simulink model "rfsoc4x2_tut_rfdc"  (R2019a)
settings: Solver=VariableStepAuto  StartTime=0.0  StopTime=10.0  RelTol=1e-3
undefined symbols (not defined in the file): I, Q
libraries: xbsIndex_r4 x704, casper_library_misc x5, xps_library x1
(part 1 of 14)
settings Model: Creator=mcb  LastModifiedBy=mcb

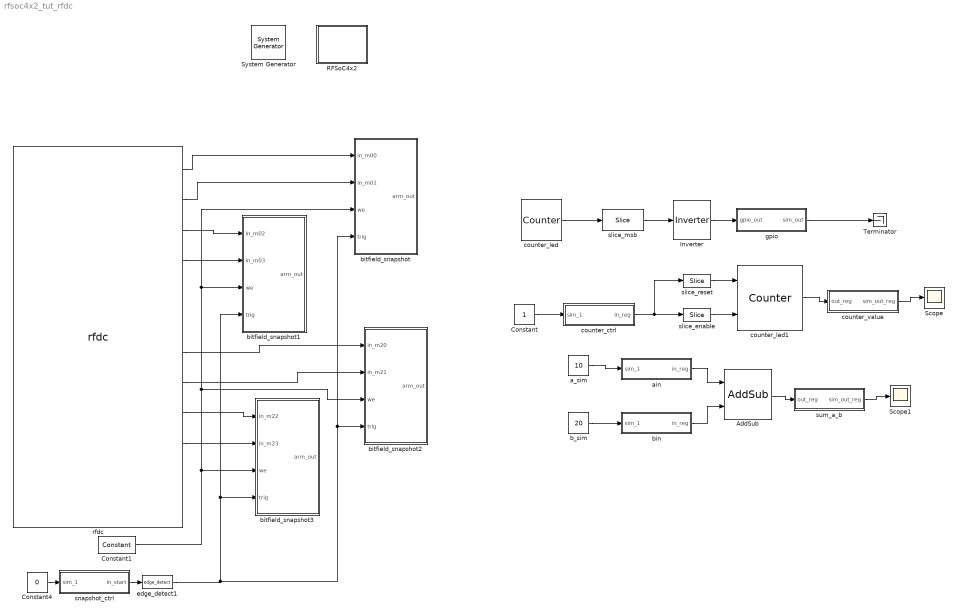
== system rfsoc4x2_tut_rfdc ==
  " System Generator" : xbsIndex_r4/ System Generator  Tag=genX  xilinxfamily=zynquplusRFSOC  part=xczu48dr  speed=-2-e  package=ffvg1517  synthesis_tool=XST  clock_wrapper=Clock Enables  directory=/home/mcb/git/casper/tutorials_devel/rfsoc/tut_rfdc/rfsoc4x2_tut_rfdc/sysgen  proj_type=Vivado  Synth_file=Vivado Synthesis Defaults  Impl_file=Vivado Implementation Defaults  testbench=off  simulink_period=1  sysclk_period=4.069  dcm_input_clock_period=10  incr_netlist=off  trim_vbits=Everywhere in SubSystem  dbl_ovrd=According to Block Masks  core_generation=According to Block Masks  run_coregen=off  deprecated_control=off  eval_field=0  block_type=sysgen
  AddSub : xbsIndex_r4/AddSub  mode=Addition  use_carryin=off  use_carryout=off  en=off  latency=0  precision=User Defined  arith_type=Unsigned  n_bits=32  bin_pt=0  quantization=Truncate  overflow=Saturate  use_behavioral_HDL=off  hw_selection=Fabric  pipelined=off  dbl_ovrd=off  block_type=addsub
  Constant : Constant
  Constant1 : xbsIndex_r4/Constant  const=1.0  gui_display_data_type=Boolean  arith_type=Boolean  n_bits=16  bin_pt=14  preci_type=Single  exp_width=8  frac_width=24  explicit_period=on  period=1  equ=P=C  opselect=C  inp2=PCIN>>17  opr=+  inp1=P  carry=CIN  dbl_ovrd=off  block_type=constant
  Constant4 : Constant  Value=0
  Inverter : xbsIndex_r4/Inverter  en=off  latency=0  dbl_ovrd=off  block_type=inv
  RFSoC4x2 : Subsystem  Tag=xps:xsg  AncestorBlock=xps_library/Platforms/ZCU216  mask(xsg core config){hw_sys=rfsoc4x2:xczu48dr, clk_src=adc_clk, clk_rate=245.76, pl_clk_rate=122.88, sample_period=1, synthesis_tool=XST}
      mask prompts: hw_sys "Hardware Platform"; clk_src "User IP Clock source"; clk_rate "User IP Clock Rate (MHz)"; pl_clk_rate "RFPLL PL Clock Rate (MHz)"; sample_period "Sample Period"; synthesis_tool "Synthesis Tool:"
      mask help:
      | The XSG Core Config block is used to configure the System Generator design
      | for the casper_xps toolflow. Settings here are used to configure the
      | Xilinx System Generator block parameters automatically, and control toolflow
      | script  execution. It needs to be at the top level of all designs being compiled
      | with the casper_xps toolflow.
      mask init:
      | xps_xsg_rfsoc4x2_conf_mask;
      mask Help: eval('xlWeb([getenv(''MLIB_ROOT''), ''\doc\html\sys_xsg_core_config\sys_xsg_core_config.html''])')
      mask TypeOptions hw_sys: rfsoc4x2:xczu48dr
      mask TypeOptions clk_src: adc_clk
      mask TypeOptions synthesis_tool: Leonardo Spectrum | Synplify | Synplify Pro | XST
      mask Display: fprintf(['RFSoC4x2']);
  Scope : Scope
  Scope1 : Scope
  Terminator : Terminator
  a_sim : Constant  Value=10
  ain : Subsystem  Tag=xps:sw_reg  AncestorBlock=xps_library/Memory/software_register  mask(swreg){io_dir=From Processor, io_delay=0, init_val=0, sample_period=1, names=reg, bitwidths=32, bin_pts=0, arith_types=0, sim_port=on, show_format=off}
      mask prompts: io_dir "I/O direction"; io_delay "I/O delay"; init_val "Initial Value"; sample_period "Sample period"; names "Bitfield names [msb...lsb]"; bitwidths "Bitfield widths"; bin_pts "Bitfield binary pts"; arith_types "Bitfield types, ufix=0, fix=1, bool=2"; sim_port "Provide sim input/output?"; show_format "Print format string?"
      mask help: A 32-bit software-accessible register. Can be divided into bitfields of varying widths and types using the fields in the block mask.
      mask init:
      | swreg_init(gcb)
      settings: AttributesFormatString=1input
      mask TypeOptions io_dir: To Processor | From Processor
      mask Callback io_dir:
      | mask_enables = get_param(gcb, 'MaskEnables');
      | mask_names = get_param(gcb, 'MaskNames');
      | if strcmp(get_param(gcb, 'io_dir'), 'To Processor'),
      |     mask_enables{ismember(mask_names, 'sample_period')} = 'off';
      | else
      |     mask_enables{ismember(mask_names, 'sample_period')} = 'on';
      | end
      | set_param(gcb, 'MaskEnables', mask_enables);
      mask DialogControl ParameterTabVar0 Prompt: Setup
  b_sim : Constant  Value=20
  bin : Subsystem  Tag=xps:sw_reg  AncestorBlock=xps_library/Memory/software_register  mask(swreg){io_dir=From Processor, io_delay=0, init_val=0, sample_period=1, names=reg, bitwidths=32, bin_pts=0, arith_types=0, sim_port=on, show_format=off}
      mask prompts: io_dir "I/O direction"; io_delay "I/O delay"; init_val "Initial Value"; sample_period "Sample period"; names "Bitfield names [msb...lsb]"; bitwidths "Bitfield widths"; bin_pts "Bitfield binary pts"; arith_types "Bitfield types, ufix=0, fix=1, bool=2"; sim_port "Provide sim input/output?"; show_format "Print format string?"
      mask help: A 32-bit software-accessible register. Can be divided into bitfields of varying widths and types using the fields in the block mask.
      mask init:
      | swreg_init(gcb)
      settings: AttributesFormatString=1input
      mask TypeOptions io_dir: To Processor | From Processor
      mask Callback io_dir:
      | mask_enables = get_param(gcb, 'MaskEnables');
      | mask_names = get_param(gcb, 'MaskNames');
      | if strcmp(get_param(gcb, 'io_dir'), 'To Processor'),
      |     mask_enables{ismember(mask_names, 'sample_period')} = 'off';
      | else
      |     mask_enables{ismember(mask_names, 'sample_period')} = 'on';
      | end
      | set_param(gcb, 'MaskEnables', mask_enables);
      mask DialogControl ParameterTabVar0 Prompt: Setup
  bitfield_snapshot : Subsystem  Tag=casper:bitsnap  AncestorBlock=casper_library_scopes/bitfield_snapshot  mask(bitsnap){io_names=[m00, m01], io_widths=[64 64], io_bps=[0 0], io_types=[1 1], show_format=on, snap_storage=bram, snap_dram_dimm=2, snap_dram_clock=250, snap_nsamples=14, snap_data_width=128, snap_offset=off, snap_circap=off, snap_value=off, snap_ext_arm=off, snap_ext_circ=off, snap_provide_outputs=on, snap_use_dsp48=on, snap_delay=2, extra_names=[c d], extra_widths=[30 2], extra_bps=[0 0], extra_types=[0 0]}
      mask prompts: io_names "Names [msb...lsb]"; io_widths "Bitwidths [msb...lsb]"; io_bps "Binary pts [msb...lsb]"; io_types "Data types [msb...lsb], ufix=0, fix=1, bool=2"; show_format "Print format string?"; snap_storage "Storage medium"; snap_dram_dimm "DRAM dimm"; snap_dram_clock "DRAM clock rate"; snap_nsamples "Number of Samples (2^?)"; snap_data_width "Data width"; snap_offset "Start delay support"; snap_circap "Circular capture support"; snap_value "Extra value capture support"; snap_ext_arm "External arm support"; snap_ext_circ "External circular capture support"; snap_provide_outputs "Provide outputs"; snap_use_dsp48 "Use DSP48s to implement counters"; snap_delay "Pre-snapshot delay"; extra_names "Names [msb...lsb]"; extra_widths "Widths [msb...lsb]"; extra_bps "Binary pts [msb...lsb]"; extra_types "Data types [msb...lsb], ufix=0, fix=1, bool=2"
      mask help:
      | A wrapped snapshot block. Allows specification of inputs to a snapblock word so the toolflow can automatically set up the scope.
      | See documentation for snapshot for explanation of parameters.
      mask init:
      | bitsnap_init(gcb);
      settings: AttributesFormatString=|
      | snap(2):f64.0,f64.0 = 128 bits\n128 wide, 16384 deep
      | debugID: 67280215
      mask TypeOptions snap_storage: bram | dram
      mask Callback snap_storage: bitsnap_callback();
      mask TypeOptions snap_dram_dimm: 1 | 2 | 3 | 4
      mask TypeOptions snap_dram_clock: 200 | 250 | 266 | 300 | 333
      mask TypeOptions snap_data_width: 8 | 16 | 32 | 64 | 128
      mask Callback snap_value: bitsnap_callback();
      mask Callback snap_ext_arm: bitsnap_callback();
      mask Callback snap_ext_circ: bitsnap_callback();
      mask Callback snap_provide_outputs: bitsnap_callback();
      mask DialogControl ParameterTabVar0 Prompt: Inputs
      mask DialogControl ParameterTabVar01 Prompt: Snapshot
      mask DialogControl ParameterTabVar012 Prompt: Extra Value
  bitfield_snapshot1 : Subsystem  Tag=casper:bitsnap  AncestorBlock=casper_library_scopes/bitfield_snapshot  mask(bitsnap){io_names=[m02, m03], io_widths=[64 64], io_bps=[0 0], io_types=[1 1], show_format=on, snap_storage=bram, snap_dram_dimm=2, snap_dram_clock=250, snap_nsamples=14, snap_data_width=128, snap_offset=off, snap_circap=off, snap_value=off, snap_ext_arm=off, snap_ext_circ=off, snap_provide_outputs=on, snap_use_dsp48=on, snap_delay=2, extra_names=[c d], extra_widths=[30 2], extra_bps=[0 0], extra_types=[0 0]}
      mask prompts: io_names "Names [msb...lsb]"; io_widths "Bitwidths [msb...lsb]"; io_bps "Binary pts [msb...lsb]"; io_types "Data types [msb...lsb], ufix=0, fix=1, bool=2"; show_format "Print format string?"; snap_storage "Storage medium"; snap_dram_dimm "DRAM dimm"; snap_dram_clock "DRAM clock rate"; snap_nsamples "Number of Samples (2^?)"; snap_data_width "Data width"; snap_offset "Start delay support"; snap_circap "Circular capture support"; snap_value "Extra value capture support"; snap_ext_arm "External arm support"; snap_ext_circ "External circular capture support"; snap_provide_outputs "Provide outputs"; snap_use_dsp48 "Use DSP48s to implement counters"; snap_delay "Pre-snapshot delay"; extra_names "Names [msb...lsb]"; extra_widths "Widths [msb...lsb]"; extra_bps "Binary pts [msb...lsb]"; extra_types "Data types [msb...lsb], ufix=0, fix=1, bool=2"
      mask help:
      | A wrapped snapshot block. Allows specification of inputs to a snapblock word so the toolflow can automatically set up the scope.
      | See documentation for snapshot for explanation of parameters.
      mask init:
      | bitsnap_init(gcb);
      settings: AttributesFormatString=|
      | snap(2):f64.0,f64.0 = 128 bits\n128 wide, 16384 deep
      | debugID: 72415094
      mask TypeOptions snap_storage: bram | dram
      mask Callback snap_storage: bitsnap_callback();
      mask TypeOptions snap_dram_dimm: 1 | 2 | 3 | 4
      mask TypeOptions snap_dram_clock: 200 | 250 | 266 | 300 | 333
      mask TypeOptions snap_data_width: 8 | 16 | 32 | 64 | 128
      mask Callback snap_value: bitsnap_callback();
      mask Callback snap_ext_arm: bitsnap_callback();
      mask Callback snap_ext_circ: bitsnap_callback();
      mask Callback snap_provide_outputs: bitsnap_callback();
      mask DialogControl ParameterTabVar0 Prompt: Inputs
      mask DialogControl ParameterTabVar01 Prompt: Snapshot
      mask DialogControl ParameterTabVar012 Prompt: Extra Value
  bitfield_snapshot2 : Subsystem  Tag=casper:bitsnap  AncestorBlock=casper_library_scopes/bitfield_snapshot  mask(bitsnap){io_names=[m20, m21], io_widths=[64 64], io_bps=[0 0], io_types=[1 1], show_format=on, snap_storage=bram, snap_dram_dimm=2, snap_dram_clock=250, snap_nsamples=14, snap_data_width=128, snap_offset=off, snap_circap=off, snap_value=off, snap_ext_arm=off, snap_ext_circ=off, snap_provide_outputs=on, snap_use_dsp48=on, snap_delay=2, extra_names=[c d], extra_widths=[30 2], extra_bps=[0 0], extra_types=[0 0]}
      mask prompts: io_names "Names [msb...lsb]"; io_widths "Bitwidths [msb...lsb]"; io_bps "Binary pts [msb...lsb]"; io_types "Data types [msb...lsb], ufix=0, fix=1, bool=2"; show_format "Print format string?"; snap_storage "Storage medium"; snap_dram_dimm "DRAM dimm"; snap_dram_clock "DRAM clock rate"; snap_nsamples "Number of Samples (2^?)"; snap_data_width "Data width"; snap_offset "Start delay support"; snap_circap "Circular capture support"; snap_value "Extra value capture support"; snap_ext_arm "External arm support"; snap_ext_circ "External circular capture support"; snap_provide_outputs "Provide outputs"; snap_use_dsp48 "Use DSP48s to implement counters"; snap_delay "Pre-snapshot delay"; extra_names "Names [msb...lsb]"; extra_widths "Widths [msb...lsb]"; extra_bps "Binary pts [msb...lsb]"; extra_types "Data types [msb...lsb], ufix=0, fix=1, bool=2"
      mask help:
      | A wrapped snapshot block. Allows specification of inputs to a snapblock word so the toolflow can automatically set up the scope.
      | See documentation for snapshot for explanation of parameters.
      mask init:
      | bitsnap_init(gcb);
      settings: AttributesFormatString=|
      | snap(2):f64.0,f64.0 = 128 bits\n128 wide, 16384 deep
      | debugID: 72444885
      mask TypeOptions snap_storage: bram | dram
      mask Callback snap_storage: bitsnap_callback();
      mask TypeOptions snap_dram_dimm: 1 | 2 | 3 | 4
      mask TypeOptions snap_dram_clock: 200 | 250 | 266 | 300 | 333
      mask TypeOptions snap_data_width: 8 | 16 | 32 | 64 | 128
      mask Callback snap_value: bitsnap_callback();
      mask Callback snap_ext_arm: bitsnap_callback();
      mask Callback snap_ext_circ: bitsnap_callback();
      mask Callback snap_provide_outputs: bitsnap_callback();
      mask DialogControl ParameterTabVar0 Prompt: Inputs
      mask DialogControl ParameterTabVar01 Prompt: Snapshot
      mask DialogControl ParameterTabVar012 Prompt: Extra Value
  bitfield_snapshot3 : Subsystem  Tag=casper:bitsnap  AncestorBlock=casper_library_scopes/bitfield_snapshot  mask(bitsnap){io_names=[m22, m23], io_widths=[64 64], io_bps=[0 0], io_types=[1 1], show_format=on, snap_storage=bram, snap_dram_dimm=2, snap_dram_clock=250, snap_nsamples=14, snap_data_width=128, snap_offset=off, snap_circap=off, snap_value=off, snap_ext_arm=off, snap_ext_circ=off, snap_provide_outputs=on, snap_use_dsp48=on, snap_delay=2, extra_names=[c d], extra_widths=[30 2], extra_bps=[0 0], extra_types=[0 0]}
      mask prompts: io_names "Names [msb...lsb]"; io_widths "Bitwidths [msb...lsb]"; io_bps "Binary pts [msb...lsb]"; io_types "Data types [msb...lsb], ufix=0, fix=1, bool=2"; show_format "Print format string?"; snap_storage "Storage medium"; snap_dram_dimm "DRAM dimm"; snap_dram_clock "DRAM clock rate"; snap_nsamples "Number of Samples (2^?)"; snap_data_width "Data width"; snap_offset "Start delay support"; snap_circap "Circular capture support"; snap_value "Extra value capture support"; snap_ext_arm "External arm support"; snap_ext_circ "External circular capture support"; snap_provide_outputs "Provide outputs"; snap_use_dsp48 "Use DSP48s to implement counters"; snap_delay "Pre-snapshot delay"; extra_names "Names [msb...lsb]"; extra_widths "Widths [msb...lsb]"; extra_bps "Binary pts [msb...lsb]"; extra_types "Data types [msb...lsb], ufix=0, fix=1, bool=2"
      mask help:
      | A wrapped snapshot block. Allows specification of inputs to a snapblock word so the toolflow can automatically set up the scope.
      | See documentation for snapshot for explanation of parameters.
      mask init:
      | bitsnap_init(gcb);
      settings: AttributesFormatString=|
      | snap(2):f64.0,f64.0 = 128 bits\n128 wide, 16384 deep
      | debugID: 72474676
      mask TypeOptions snap_storage: bram | dram
      mask Callback snap_storage: bitsnap_callback();
      mask TypeOptions snap_dram_dimm: 1 | 2 | 3 | 4
      mask TypeOptions snap_dram_clock: 200 | 250 | 266 | 300 | 333
      mask TypeOptions snap_data_width: 8 | 16 | 32 | 64 | 128
      mask Callback snap_value: bitsnap_callback();
      mask Callback snap_ext_arm: bitsnap_callback();
      mask Callback snap_ext_circ: bitsnap_callback();
      mask Callback snap_provide_outputs: bitsnap_callback();
      mask DialogControl ParameterTabVar0 Prompt: Inputs
      mask DialogControl ParameterTabVar01 Prompt: Snapshot
      mask DialogControl ParameterTabVar012 Prompt: Extra Value
  counter_ctrl : Subsystem  Tag=xps:sw_reg  AncestorBlock=xps_library/Memory/software_register  mask(swreg){io_dir=From Processor, io_delay=0, init_val=0, sample_period=1, names=reg, bitwidths=32, bin_pts=0, arith_types=0, sim_port=on, show_format=off}
      mask prompts: io_dir "I/O direction"; io_delay "I/O delay"; init_val "Initial Value"; sample_period "Sample period"; names "Bitfield names [msb...lsb]"; bitwidths "Bitfield widths"; bin_pts "Bitfield binary pts"; arith_types "Bitfield types, ufix=0, fix=1, bool=2"; sim_port "Provide sim input/output?"; show_format "Print format string?"
      mask help: A 32-bit software-accessible register. Can be divided into bitfields of varying widths and types using the fields in the block mask.
      mask init:
      | swreg_init(gcb)
      settings: AttributesFormatString=1input
      mask TypeOptions io_dir: To Processor | From Processor
      mask Callback io_dir:
      | mask_enables = get_param(gcb, 'MaskEnables');
      | mask_names = get_param(gcb, 'MaskNames');
      | if strcmp(get_param(gcb, 'io_dir'), 'To Processor'),
      |     mask_enables{ismember(mask_names, 'sample_period')} = 'off';
      | else
      |     mask_enables{ismember(mask_names, 'sample_period')} = 'on';
      | end
      | set_param(gcb, 'MaskEnables', mask_enables);
      mask DialogControl ParameterTabVar0 Prompt: Setup
  counter_led : xbsIndex_r4/Counter  cnt_type=Free Running  cnt_to=Inf  operation=Up  start_count=0  cnt_by_val=1  arith_type=Unsigned  n_bits=28  bin_pt=0  load_pin=off  rst=off  en=off  explicit_period=on  period=1  use_behavioral_HDL=off  implementation=Fabric  dbl_ovrd=off  block_type=counter
  counter_led1 : xbsIndex_r4/Counter  cnt_type=Free Running  cnt_to=Inf  operation=Up  start_count=0  cnt_by_val=1  arith_type=Unsigned  n_bits=32  bin_pt=0  load_pin=off  rst=on  en=on  explicit_period=on  period=1  use_behavioral_HDL=off  implementation=Fabric  dbl_ovrd=off  block_type=counter
  counter_value : Subsystem  Tag=xps:sw_reg  AncestorBlock=xps_library/Memory/software_register  mask(swreg){io_dir=To Processor, io_delay=0, init_val=0, sample_period=1, names=reg, bitwidths=32, bin_pts=0, arith_types=0, sim_port=on, show_format=off}
      mask prompts: io_dir "I/O direction"; io_delay "I/O delay"; init_val "Initial Value"; sample_period "Sample period"; names "Bitfield names [msb...lsb]"; bitwidths "Bitfield widths"; bin_pts "Bitfield binary pts"; arith_types "Bitfield types, ufix=0, fix=1, bool=2"; sim_port "Provide sim input/output?"; show_format "Print format string?"
      mask help: A 32-bit software-accessible register. Can be divided into bitfields of varying widths and types using the fields in the block mask.
      mask init:
      | swreg_init(gcb)
      settings: AttributesFormatString=1output
      mask TypeOptions io_dir: To Processor | From Processor
      mask Callback io_dir:
      | mask_enables = get_param(gcb, 'MaskEnables');
      | mask_names = get_param(gcb, 'MaskNames');
      | if strcmp(get_param(gcb, 'io_dir'), 'To Processor'),
      |     mask_enables{ismember(mask_names, 'sample_period')} = 'off';
      | else
      |     mask_enables{ismember(mask_names, 'sample_period')} = 'on';
      | end
      | set_param(gcb, 'MaskEnables', mask_enables);
      mask DialogControl ParameterTabVar0 Prompt: Setup
  edge_detect1 : casper_library_misc/edge_detect  edge=Rising  polarity=Active High  x_in=[0 0.08 0.08 0.16 0.16 0.24 0.24 0.32 0.32 0.4]  y_in="[-1 -1  1  1  1  1  1  1  1  1]"  x_out=[0.6 0.68 0.68 0.76 0.76 0.84 0.84 0.92 0.92 1]  y_out="[-1 -1  1  1 -1 -1 -1 -1 -1 -1]"
  gpio : Subsystem  Tag=xps:gpio  AncestorBlock=xps_library/IO/gpio  mask(gpio){io_group_params_forwarded=on, io_group=ROACH2:led, io_group_real=led, io_group_custom=0, io_dir=out, arith_type=Boolean, bitwidth=1, bin_pt=0, bit_index=0, sample_period=1, use_single_ended=off, use_ddr=off, reg_iob=on, reg_clk_phase=0, termination=None}
      mask prompts: io_group_params_forwarded "Have the io_group params been forwarded yet?"; io_group "I/O group"; io_group_real "I/O group"; io_group_custom "Custom I/O group"; io_dir "I/O direction"; arith_type "Data Type"; bitwidth "Data bitwidth"; bin_pt "Data binary point"; bit_index "GPIO bit index"; sample_period "Sample period"; use_single_ended "Use as single-ended"; use_ddr "Use DDR"; reg_iob "Pack register in the pad"; reg_clk_phase "Register clock phase"; termination "Termination method"
      mask help:
      | GPIO interfaces for CASPER hardware.
      |
      | For usage of LEDs on SKARAB boards, please note that the board will boot into 'BSP mode' by default. To change the control of the Front Panel LEDs to your design, execute the command 'control_front_panel_leds_write()' on your SKARAB CASPERFPGA object via the transport layer.
      |
      | For more information please click help below.
      mask init:
      | gpio_mask;
      mask Help: If you've come here for more help, unfortunately I'm going to direct you to the ska-sa/casperfpga wiki. The documentation at https://github.com/ska-sa/casperfpga/wiki/SKARAB-Front-Panel-LED-Manager outlines the signals that are used to control the SKARAB's Front Panel LEDs by default, and the mechanism by which you can switch control to the DSP Design.
      mask TypeOptions io_group: ROACH:aux0_clk | ROACH:aux1_clk | ROACH:led | ROACH:gpioa | ROACH:gpioa_oe_n | ROACH:gpiob | ROACH:gpiob_oe_n | ROACH:qsh | ROACH:zdok0 | ROACH:zdok1 | ROACH2:aux_clk | ROACH2:led | ROACH2:gpio | ROACH2:qsh | ROACH2:sync_in | ROACH2:sync_out | ROACH2:zdok0 | ROACH2:zdok1 | custom:custom
      mask TypeOptions io_group_real: led | gpio | sync_in | sync_out | zdok0 | zdok1 | aux_clk_diff | custom
      mask Callback io_group_real:
      | if ~isempty(find(strcmp(get_param(gcb, 'io_group_real'), {'zdok0' 'zdok1' 'sync_in' 'sync_out'})))
      |     set_param(gcb, 'MaskEnables', {'off', 'off', 'on','off','on','on','on','on','on','on','on','on','on','on','on'});
      | elseif ~isempty(find(strcmp(get_param(gcb, 'io_group_real'), {'custom'})))
      |     set_param(gcb, 'MaskEnables', {'off', 'off', 'on','on','on','on','on','on','on','on','off','on','on','on','on'});
      | else
      |     set_param(gcb, 'MaskEnables', {'off', 'off', 'on','off','on','on','on','on','on','on','off','on','on','on','on'});
      | end
      mask TypeOptions io_dir: in | out
      mask Callback io_dir:
      | if ~isempty(find(strcmp(get_param(gcb, 'io_group_real'), {'zdok0' 'zdok1' 'sync_in' 'sync_out'})))
      |     set_param(gcb, 'MaskVisibilities', {'off', 'off','on','on','on','on','on','on','on','on','on','on','on','on','on'});
      | else
      |     set_param(gcb, 'MaskVisibilities', {'off', 'off','on','on','on','on','on','on','on','on','off','on','on','on','on'});
      | end
      mask TypeOptions arith_type: Boolean | Unsigned | Signed  (2's comp)
      mask Callback use_ddr:
      | if strcmp(get_param(gcb,'use_ddr'),'on')
      |     set_param(gcb,'reg_iob','on');
      |     set_param(gcb,'MaskEnables', {'off' 'off' 'on' 'on' 'on' 'on' 'on' 'on' 'on' 'on' 'on' 'on' 'off' 'on' 'on'});
      | else
      |     set_param(gcb,'MaskEnables', {'off' 'off' 'on' 'on' 'on' 'on' 'on' 'on' 'on' 'on' 'on' 'on' 'on' 'on' 'on'});
      | end
      mask TypeOptions reg_clk_phase: 0 | 90 | 180 | 270
      mask TypeOptions termination: None | Pullup | Pulldown
  rfdc : xps_library/ADCs/rfdc  Tag=xps:rfdc  forceredraw=0  maskopening=1  runinit=1  Tile224_enable=on  t224_enable_mts=off  t224_sample_rate=3932.16  t224_clk_out=245.76  t224_enable_pll=on  t224_ref_clk=491.52  t224_QT_adc0_enable=on  t224_QT_adc0_digital_output=I/Q  t224_QT_adc0_dec_mode=4x  t224_QT_adc0_sample_per_cycle=4  t224_QT_adc0_req_axis_clk=250  t224_QT_adc0_mixer_type=Fine  t224_QT_adc0_mixer_mode=Real -> I/Q  t224_QT_adc0_nco_freq=0  t224_QT_adc0_nco_phase=0  t224_QT_adc0_coarse_freq=0  t224_QT_adc0_nyquist_zone=Zone 1  t224_QT_adc0_cal_mode=Mode 2  t224_QT_adc1_enable=on  t224_QT_adc1_digital_output=I/Q  t224_QT_adc1_dec_mode=4x  t224_QT_adc1_sample_per_cycle=4  t224_QT_adc1_req_axis_clk=250  t224_QT_adc1_mixer_type=Fine  t224_QT_adc1_mixer_mode=Real -> I/Q  t224_QT_adc1_nco_freq=0  t224_QT_adc1_nco_phase=0  t224_QT_adc1_coarse_freq=0  t224_QT_adc1_nyquist_zone=Zone 1  t224_QT_adc1_cal_mode=Mode 2  t224_QT_adc2_enable=on  t224_QT_adc2_digital_output=I/Q  t224_QT_adc2_dec_mode=4x  t224_QT_adc2_sample_per_cycle=4  t224_QT_adc2_req_axis_clk=250  t224_QT_adc2_mixer_type=Fine  t224_QT_adc2_mixer_mode=Real -> I/Q  t224_QT_adc2_nco_freq=0  t224_QT_adc2_nco_phase=0  t224_QT_adc2_coarse_freq=0  t224_QT_adc2_nyquist_zone=Zone 1  t224_QT_adc2_cal_mode=Mode 2  t224_QT_adc3_enable=on  t224_QT_adc3_digital_output=I/Q  t224_QT_adc3_dec_mode=4x  t224_QT_adc3_sample_per_cycle=4  t224_QT_adc3_req_axis_clk=250  t224_QT_adc3_mixer_type=Fine  t224_QT_adc3_mixer_mode=Real -> I/Q  t224_QT_adc3_nco_freq=0  t224_QT_adc3_nco_phase=0  t224_QT_adc3_coarse_freq=0  t224_QT_adc3_nyquist_zone=Zone 1  t224_QT_adc3_cal_mode=Mode 2  t224_DT_adc0_enable=on  t224_DT_adc0_digital_output=I/Q  t224_DT_adc0_dec_mode=4x  t224_DT_adc0_sample_per_cycle=4  t224_DT_adc0_req_axis_clk=245.76  t224_DT_adc0_mixer_type=Fine  t224_DT_adc0_mixer_mode=Real -> I/Q  t224_DT_adc0_nco_freq=-1.5  t224_DT_adc0_nco_phase=0  t224_DT_adc0_coarse_freq=0  t224_DT_adc0_nyquist_zone=Zone 1  t224_DT_adc0_cal_mode=Mode 2  t224_DT_adc1_enable=on  t224_DT_adc1_digital_output=I/Q  t224_DT_adc1_dec_mode=4x  t224_DT_adc1_sample_per_cycle=4  t224_DT_adc1_req_axis_clk=245.76  t224_DT_adc1_mixer_type=Fine  t224_DT_adc1_mixer_mode=Real -> I/Q  t224_DT_adc1_nco_freq=-1.5  t224_DT_adc1_nco_phase=0  t224_DT_adc1_coarse_freq=0  t224_DT_adc1_nyquist_zone=Zone 1  t224_DT_adc1_cal_mode=Mode 2  Tile225_enable=on  t225_enable_mts=off  t225_sample_rate=3932.16  t225_clk_out=245.76  t225_enable_pll=on  t225_ref_clk=491.52  t225_QT_adc0_enable=on  t225_QT_adc0_digital_output=Real  t225_QT_adc0_dec_mode=4x  t225_QT_adc0_sample_per_cycle=2  t225_QT_adc0_req_axis_clk=250  t225_QT_adc0_mixer_type=Bypassed  t225_QT_adc0_mixer_mode=Real -> Real  t225_QT_adc0_nco_freq=0  t225_QT_adc0_nco_phase=0  t225_QT_adc0_coarse_freq=0  t225_QT_adc0_nyquist_zone=Zone 1  t225_QT_adc0_cal_mode=Mode 2  t225_QT_adc1_enable=off  t225_QT_adc1_digital_output=Real  t225_QT_adc1_dec_mode=4x  t225_QT_adc1_sample_per_cycle=2  t225_QT_adc1_req_axis_clk=250  t225_QT_adc1_mixer_type=Bypassed  t225_QT_adc1_mixer_mode=Real -> Real  t225_QT_adc1_nco_freq=0  t225_QT_adc1_nco_phase=0  t225_QT_adc1_coarse_freq=0  t225_QT_adc1_nyquist_zone=Zone 1  t225_QT_adc1_cal_mode=Mode 2  t225_QT_adc2_enable=off  t225_QT_adc2_digital_output=Real  t225_QT_adc2_dec_mode=4x  t225_QT_adc2_sample_per_cycle=2  t225_QT_adc2_req_axis_clk=250  t225_QT_adc2_mixer_type=Bypassed  t225_QT_adc2_mixer_mode=Real -> Real  t225_QT_adc2_nco_freq=0  t225_QT_adc2_nco_phase=0  t225_QT_adc2_coarse_freq=0  t225_QT_adc2_nyquist_zone=Zone 1  t225_QT_adc2_cal_mode=Mode 2  t225_QT_adc3_enable=off  t225_QT_adc3_digital_output=Real  t225_QT_adc3_dec_mode=4x  t225_QT_adc3_sample_per_cycle=2  t225_QT_adc3_req_axis_clk=250  t225_QT_adc3_mixer_type=Bypassed  t225_QT_adc3_mixer_mode=Real -> Real  t225_QT_adc3_nco_freq=0  t225_QT_adc3_nco_phase=0  t225_QT_adc3_coarse_freq=0  t225_QT_adc3_nyquist_zone=Zone 1  t225_QT_adc3_cal_mode=Mode 2  t225_DT_adc0_enable=on  t225_DT_adc0_digital_output=Real  t225_DT_adc0_dec_mode=2x  t225_DT_adc0_sample_per_cycle=8  t225_DT_adc0_req_axis_clk=245.76  t225_DT_adc0_mixer_type=Bypassed  t225_DT_adc0_mixer_mode=Real -> Real  t225_DT_adc0_nco_freq=0  t225_DT_adc0_nco_phase=0  t225_DT_adc0_coarse_freq=0  t225_DT_adc0_nyquist_zone=Zone 1  t225_DT_adc0_cal_mode=Mode 2  t225_DT_adc1_enable=on  t225_DT_adc1_digital_output=Real  t225_DT_adc1_dec_mode=2x  t225_DT_adc1_sample_per_cycle=8  t225_DT_adc1_req_axis_clk=245.76  t225_DT_adc1_mixer_type=Bypassed  t225_DT_adc1_mixer_mode=Real -> Real  t225_DT_adc1_nco_freq=0  t225_DT_adc1_nco_phase=0  t225_DT_adc1_coarse_freq=0  t225_DT_adc1_nyquist_zone=Zone 1  t225_DT_adc1_cal_mode=Mode 2  Tile226_enable=on  t226_enable_mts=off  t226_sample_rate=3932.16  t226_clk_out=245.76  t226_enable_pll=on  t226_ref_clk=491.52  t226_QT_adc0_enable=on  t226_QT_adc0_digital_output=Real  t226_QT_adc0_dec_mode=4x  t226_QT_adc0_sample_per_cycle=2  t226_QT_adc0_req_axis_clk=250  t226_QT_adc0_mixer_type=Bypassed  t226_QT_adc0_mixer_mode=Real -> Real  t226_QT_adc0_nco_freq=0  t226_QT_adc0_nco_phase=0  t226_QT_adc0_coarse_freq=0  t226_QT_adc0_nyquist_zone=Zone 1  t226_QT_adc0_cal_mode=Mode 2  t226_QT_adc1_enable=off  t226_QT_adc1_digital_output=Real  t226_QT_adc1_dec_mode=4x  t226_QT_adc1_sample_per_cycle=2  t226_QT_adc1_req_axis_clk=250  t226_QT_adc1_mixer_type=Bypassed  t226_QT_adc1_mixer_mode=Real -> Real  t226_QT_adc1_nco_freq=0  t226_QT_adc1_nco_phase=0  t226_QT_adc1_coarse_freq=0  t226_QT_adc1_nyquist_zone=Zone 1  t226_QT_adc1_cal_mode=Mode 2  t226_QT_adc2_enable=off  t226_QT_adc2_digital_output=Real  t226_QT_adc2_dec_mode=4x  t226_QT_adc2_sample_per_cycle=2  t226_QT_adc2_req_axis_clk=250  t226_QT_adc2_mixer_type=Bypassed  t226_QT_adc2_mixer_mode=Real -> Real  t226_QT_adc2_nco_freq=0  t226_QT_adc2_nco_phase=0  t226_QT_adc2_coarse_freq=0  t226_QT_adc2_nyquist_zone=Zone 1  t226_QT_adc2_cal_mode=Mode 2  t226_QT_adc3_enable=off  t226_QT_adc3_digital_output=Real  t226_QT_adc3_dec_mode=4x  t226_QT_adc3_sample_per_cycle=2  t226_QT_adc3_req_axis_clk=250  t226_QT_adc3_mixer_type=Bypassed  t226_QT_adc3_mixer_mode=Real -> Real  t226_QT_adc3_nco_freq=0  t226_QT_adc3_nco_phase=0  t226_QT_adc3_coarse_freq=0  t226_QT_adc3_nyquist_zone=Zone 1  t226_QT_adc3_cal_mode=Mode 2  t226_DT_adc0_enable=on  t226_DT_adc0_digital_output=I/Q  t226_DT_adc0_dec_mode=4x  t226_DT_adc0_sample_per_cycle=4  t226_DT_adc0_req_axis_clk=245.76  t226_DT_adc0_mixer_type=Fine  t226_DT_adc0_mixer_mode=Real -> I/Q  t226_DT_adc0_nco_freq=-1.5  t226_DT_adc0_nco_phase=0  t226_DT_adc0_coarse_freq=0  t226_DT_adc0_nyquist_zone=Zone 1  t226_DT_adc0_cal_mode=Mode 2  t226_DT_adc1_enable=on  t226_DT_adc1_digital_output=I/Q  t226_DT_adc1_dec_mode=4x  t226_DT_adc1_sample_per_cycle=4  t226_DT_adc1_req_axis_clk=245.76  t226_DT_adc1_mixer_type=Fine  t226_DT_adc1_mixer_mode=Real -> I/Q  t226_DT_adc1_nco_freq=-1.5  t226_DT_adc1_nco_phase=0  t226_DT_adc1_coarse_freq=0  t226_DT_adc1_nyquist_zone=Zone 1  t226_DT_adc1_cal_mode=Mode 2  Tile227_enable=on  t227_enable_mts=off  t227_sample_rate=3932.16  t227_clk_out=245.76  t227_enable_pll=on  t227_ref_clk=491.52  t227_QT_adc0_enable=on  t227_QT_adc0_digital_output=Real  t227_QT_adc0_dec_mode=4x  t227_QT_adc0_sample_per_cycle=2  t227_QT_adc0_req_axis_clk=250  t227_QT_adc0_mixer_type=Bypassed  t227_QT_adc0_mixer_mode=Real -> Real  t227_QT_adc0_nco_freq=0  t227_QT_adc0_nco_phase=0  t227_QT_adc0_coarse_freq=0  t227_QT_adc0_nyquist_zone=Zone 1  t227_QT_adc0_cal_mode=Mode 2  t227_QT_adc1_enable=off  t227_QT_adc1_digital_output=Real  t227_QT_adc1_dec_mode=4x  t227_QT_adc1_sample_per_cycle=2  t227_QT_adc1_req_axis_clk=250  t227_QT_adc1_mixer_type=Bypassed  t227_QT_adc1_mixer_mode=Real -> Real  t227_QT_adc1_nco_freq=0  t227_QT_adc1_nco_phase=0  t227_QT_adc1_coarse_freq=0  t227_QT_adc1_nyquist_zone=Zone 1  t227_QT_adc1_cal_mode=Mode 2  t227_QT_adc2_enable=off  t227_QT_adc2_digital_output=Real  t227_QT_adc2_dec_mode=4x  t227_QT_adc2_sample_per_cycle=2  t227_QT_adc2_req_axis_clk=250  t227_QT_adc2_mixer_type=Bypassed  t227_QT_adc2_mixer_mode=Real -> Real  t227_QT_adc2_nco_freq=0  t227_QT_adc2_nco_phase=0  t227_QT_adc2_coarse_freq=0  t227_QT_adc2_nyquist_zone=Zone 1  t227_QT_adc2_cal_mode=Mode 2  t227_QT_adc3_enable=off  t227_QT_adc3_digital_output=Real  t227_QT_adc3_dec_mode=4x  t227_QT_adc3_sample_per_cycle=2  t227_QT_adc3_req_axis_clk=250  t227_QT_adc3_mixer_type=Bypassed  t227_QT_adc3_mixer_mode=Real -> Real  t227_QT_adc3_nco_freq=0  t227_QT_adc3_nco_phase=0  t227_QT_adc3_coarse_freq=0  t227_QT_adc3_nyquist_zone=Zone 1  t227_QT_adc3_cal_mode=Mode 2  t227_DT_adc0_enable=on  t227_DT_adc0_digital_output=Real  t227_DT_adc0_dec_mode=2x  t227_DT_adc0_sample_per_cycle=8  t227_DT_adc0_req_axis_clk=245.76  t227_DT_adc0_mixer_type=Bypassed  t227_DT_adc0_mixer_mode=Real -> Real  t227_DT_adc0_nco_freq=0  t227_DT_adc0_nco_phase=0  t227_DT_adc0_coarse_freq=0  t227_DT_adc0_nyquist_zone=Zone 1  t227_DT_adc0_cal_mode=Mode 2  t227_DT_adc1_enable=on  t227_DT_adc1_digital_output=Real  t227_DT_adc1_dec_mode=2x  t227_DT_adc1_sample_per_cycle=8  t227_DT_adc1_req_axis_clk=245.76  t227_DT_adc1_mixer_type=Bypassed  t227_DT_adc1_mixer_mode=Real -> Real  t227_DT_adc1_nco_freq=0  t227_DT_adc1_nco_phase=0  t227_DT_adc1_coarse_freq=0  t227_DT_adc1_nyquist_zone=Zone 1  t227_DT_adc1_cal_mode=Mode 2  Tile228_enable=off  t228_enable_mts=off  t228_sample_rate=2000  t228_clk_out=125  t228_enable_pll=on  t228_ref_clk=250  t228_output_power=20  t228_QT_dac0_enable=on  t228_QT_dac0_analog_output=Real  t228_QT_dac0_inter_mode=4x  t228_QT_dac0_sample_per_cycle=2  t228_QT_dac0_req_axis_clk=250  t228_QT_dac0_datapath_mode=DUC 0 to Fs/2  t228_QT_dac0_mixer_type=Bypassed  t228_QT_dac0_mixer_mode=Real -> Real  t228_QT_dac0_nco_freq=0  t228_QT_dac0_nco_phase=0  t228_QT_dac0_coarse_freq=0  t228_QT_dac0_nyquist_zone=Zone 1  t228_QT_dac0_decode_mode=SNR Optimized  t228_QT_dac1_enable=on  t228_QT_dac1_analog_output=Real  t228_QT_dac1_inter_mode=4x  t228_QT_dac1_sample_per_cycle=2  t228_QT_dac1_req_axis_clk=250  t228_QT_dac1_datapath_mode=DUC 0 to Fs/2  t228_QT_dac1_mixer_type=Bypassed  t228_QT_dac1_mixer_mode=Real -> Real  t228_QT_dac1_nco_freq=0  t228_QT_dac1_nco_phase=0  t228_QT_dac1_coarse_freq=0  t228_QT_dac1_nyquist_zone=Zone 1  t228_QT_dac1_decode_mode=SNR Optimized  t228_QT_dac2_enable=off  t228_QT_dac2_analog_output=Real  t228_QT_dac2_inter_mode=4x  t228_QT_dac2_sample_per_cycle=2  t228_QT_dac2_req_axis_clk=250  t228_QT_dac2_datapath_mode=DUC 0 to Fs/2  t228_QT_dac2_mixer_type=Bypassed  t228_QT_dac2_mixer_mode=Real -> Real  t228_QT_dac2_nco_freq=0  t228_QT_dac2_nco_phase=0  t228_QT_dac2_coarse_freq=0  t228_QT_dac2_nyquist_zone=Zone 1  t228_QT_dac2_decode_mode=SNR Optimized  t228_QT_dac3_enable=off  t228_QT_dac3_analog_output=Real  t228_QT_dac3_inter_mode=4x  t228_QT_dac3_sample_per_cycle=2  t228_QT_dac3_req_axis_clk=250  t228_QT_dac3_datapath_mode=DUC 0 to Fs/2  t228_QT_dac3_mixer_type=Bypassed  t228_QT_dac3_mixer_mode=Real -> Real  t228_QT_dac3_nco_freq=0  t228_QT_dac3_nco_phase=0  t228_QT_dac3_coarse_freq=0  t228_QT_dac3_nyquist_zone=Zone 1  t228_QT_dac3_decode_mode=SNR Optimized  t228_DT_dac0_enable=off  t228_DT_dac0_analog_output=I/Q  t228_DT_dac0_inter_mode=2x  t228_DT_dac0_sample_per_cycle=8  t228_DT_dac0_req_axis_clk=250  t228_DT_dac0_mixer_type=Fine  t228_DT_dac0_mixer_mode=I/Q -> I/Q  t228_DT_dac0_nco_freq=0  t228_DT_dac0_nco_phase=0  t228_DT_dac0_coarse_freq=0  t228_DT_dac0_nyquist_zone=Zone 1  t228_DT_dac0_decode_mode=SNR Optimized  t228_DT_dac1_enable=on  t228_DT_dac1_analog_output=I/Q  t228_DT_dac1_inter_mode=2x  t228_DT_dac1_sample_per_cycle=8  t228_DT_dac1_req_axis_clk=250  t228_DT_dac1_mixer_type=Off  t228_DT_dac1_mixer_mode=I/Q -> I/Q  t228_DT_dac1_nco_freq=0  t228_DT_dac1_nco_phase=0  t228_DT_dac1_coarse_freq=0  t228_DT_dac1_nyquist_zone=Zone 1  t228_DT_dac1_decode_mode=SNR Optimized  t228_DT_dac2_enable=off  t228_DT_dac2_analog_output=Real  t228_DT_dac2_inter_mode=2x  t228_DT_dac2_sample_per_cycle=8  t228_DT_dac2_req_axis_clk=125  t228_DT_dac2_mixer_type=Bypassed  t228_DT_dac2_mixer_mode=Real -> Real  t228_DT_dac2_nco_freq=0  t228_DT_dac2_nco_phase=0  t228_DT_dac2_coarse_freq=0  t228_DT_dac2_nyquist_zone=Zone 1  t228_DT_dac2_decode_mode=SNR Optimized  t228_DT_dac3_enable=off  t228_DT_dac3_analog_output=Real  t228_DT_dac3_inter_mode=2x  t228_DT_dac3_sample_per_cycle=8  t228_DT_dac3_req_axis_clk=125  t228_DT_dac3_mixer_type=Bypassed  t228_DT_dac3_mixer_mode=Real -> Real  t228_DT_dac3_nco_freq=0  t228_DT_dac3_nco_phase=0  t228_DT_dac3_coarse_freq=0  t228_DT_dac3_nyquist_zone=Zone 1  t228_DT_dac3_decode_mode=SNR Optimized  Tile229_enable=off  t229_enable_mts=off  t229_sample_rate=2000  t229_clk_out=125  t229_enable_pll=on  t229_ref_clk=250  t229_output_power=20  t229_QT_dac0_enable=on  t229_QT_dac0_analog_output=Real  t229_QT_dac0_inter_mode=4x  t229_QT_dac0_sample_per_cycle=2  t229_QT_dac0_req_axis_clk=250  t229_QT_dac0_datapath_mode=DUC 0 to Fs/2  t229_QT_dac0_mixer_type=Bypassed  t229_QT_dac0_mixer_mode=Real -> Real  t229_QT_dac0_nco_freq=0  t229_QT_dac0_nco_phase=0  t229_QT_dac0_coarse_freq=0  t229_QT_dac0_nyquist_zone=Zone 1  t229_QT_dac0_decode_mode=SNR Optimized  t229_QT_dac1_enable=off  t229_QT_dac1_analog_output=Real  t229_QT_dac1_inter_mode=4x  t229_QT_dac1_sample_per_cycle=2  t229_QT_dac1_req_axis_clk=250  t229_QT_dac1_datapath_mode=DUC 0 to Fs/2  t229_QT_dac1_mixer_type=Bypassed  t229_QT_dac1_mixer_mode=Real -> Real  t229_QT_dac1_nco_freq=0  t229_QT_dac1_nco_phase=0  t229_QT_dac1_coarse_freq=0  t229_QT_dac1_nyquist_zone=Zone 1  t229_QT_dac1_decode_mode=SNR Optimized  t229_QT_dac2_enable=off  t229_QT_dac2_analog_output=Real  t229_QT_dac2_inter_mode=4x  t229_QT_dac2_sample_per_cycle=2  t229_QT_dac2_req_axis_clk=250  t229_QT_dac2_datapath_mode=DUC 0 to Fs/2  t229_QT_dac2_mixer_type=Bypassed  t229_QT_dac2_mixer_mode=Real -> Real  t229_QT_dac2_nco_freq=0  t229_QT_dac2_nco_phase=0  t229_QT_dac2_coarse_freq=0  t229_QT_dac2_nyquist_zone=Zone 1  t229_QT_dac2_decode_mode=SNR Optimized  t229_QT_dac3_enable=off  t229_QT_dac3_analog_output=Real  t229_QT_dac3_inter_mode=4x  t229_QT_dac3_sample_per_cycle=2  t229_QT_dac3_req_axis_clk=250  t229_QT_dac3_datapath_mode=DUC 0 to Fs/2  t229_QT_dac3_mixer_type=Bypassed  t229_QT_dac3_mixer_mode=Real -> Real  t229_QT_dac3_nco_freq=0  t229_QT_dac3_nco_phase=0  t229_QT_dac3_coarse_freq=0  t229_QT_dac3_nyquist_zone=Zone 1  t229_QT_dac3_decode_mode=SNR Optimized  t229_DT_dac0_enable=off  t229_DT_dac0_analog_output=Real  t229_DT_dac0_inter_mode=2x  t229_DT_dac0_sample_per_cycle=8  t229_DT_dac0_req_axis_clk=125  t229_DT_dac0_mixer_type=Bypassed  t229_DT_dac0_mixer_mode=Real -> Real  t229_DT_dac0_nco_freq=0  t229_DT_dac0_nco_phase=0  t229_DT_dac0_coarse_freq=0  t229_DT_dac0_nyquist_zone=Zone 1  t229_DT_dac0_decode_mode=SNR Optimized  t229_DT_dac1_enable=off  t229_DT_dac1_analog_output=Real  t229_DT_dac1_inter_mode=2x  t229_DT_dac1_sample_per_cycle=8  t229_DT_dac1_req_axis_clk=125  t229_DT_dac1_mixer_type=Bypassed  t229_DT_dac1_mixer_mode=Real -> Real  t229_DT_dac1_nco_freq=0  t229_DT_dac1_nco_phase=0  t229_DT_dac1_coarse_freq=0  t229_DT_dac1_nyquist_zone=Zone 1  t229_DT_dac1_decode_mode=SNR Optimized  t229_DT_dac2_enable=off  t229_DT_dac2_analog_output=Real  t229_DT_dac2_inter_mode=2x  t229_DT_dac2_sample_per_cycle=8  t229_DT_dac2_req_axis_clk=125  t229_DT_dac2_mixer_type=Bypassed  t229_DT_dac2_mixer_mode=Real -> Real  t229_DT_dac2_nco_freq=0  t229_DT_dac2_nco_phase=0  t229_DT_dac2_coarse_freq=0  t229_DT_dac2_nyquist_zone=Zone 1  t229_DT_dac2_decode_mode=SNR Optimized  t229_DT_dac3_enable=off  t229_DT_dac3_analog_output=Real  t229_DT_dac3_inter_mode=2x  t229_DT_dac3_sample_per_cycle=8  t229_DT_dac3_req_axis_clk=125  t229_DT_dac3_mixer_type=Bypassed  t229_DT_dac3_mixer_mode=Real -> Real  t229_DT_dac3_nco_freq=0  t229_DT_dac3_nco_phase=0  t229_DT_dac3_coarse_freq=0  t229_DT_dac3_nyquist_zone=Zone 1  t229_DT_dac3_decode_mode=SNR Optimized  Tile230_enable=off  t230_enable_mts=off  t230_sample_rate=2000  t230_clk_out=125  t230_enable_pll=on  t230_ref_clk=250  t230_output_power=20  t230_QT_dac0_enable=on  t230_QT_dac0_analog_output=Real  t230_QT_dac0_inter_mode=4x  t230_QT_dac0_sample_per_cycle=2  t230_QT_dac0_req_axis_clk=250  t230_QT_dac0_datapath_mode=DUC 0 to Fs/2  t230_QT_dac0_mixer_type=Bypassed  t230_QT_dac0_mixer_mode=Real -> Real  t230_QT_dac0_nco_freq=0  t230_QT_dac0_nco_phase=0  t230_QT_dac0_coarse_freq=0  t230_QT_dac0_nyquist_zone=Zone 1  t230_QT_dac0_decode_mode=SNR Optimized  t230_QT_dac1_enable=off  t230_QT_dac1_analog_output=Real  t230_QT_dac1_inter_mode=4x  t230_QT_dac1_sample_per_cycle=2  t230_QT_dac1_req_axis_clk=250  t230_QT_dac1_datapath_mode=DUC 0 to Fs/2  t230_QT_dac1_mixer_type=Bypassed  t230_QT_dac1_mixer_mode=Real -> Real  t230_QT_dac1_nco_freq=0  t230_QT_dac1_nco_phase=0  t230_QT_dac1_coarse_freq=0  t230_QT_dac1_nyquist_zone=Zone 1  t230_QT_dac1_decode_mode=SNR Optimized  t230_QT_dac2_enable=off  t230_QT_dac2_analog_output=Real  t230_QT_dac2_inter_mode=4x  t230_QT_dac2_sample_per_cycle=2  t230_QT_dac2_req_axis_clk=250  t230_QT_dac2_datapath_mode=DUC 0 to Fs/2  t230_QT_dac2_mixer_type=Bypassed  t230_QT_dac2_mixer_mode=Real -> Real  t230_QT_dac2_nco_freq=0  t230_QT_dac2_nco_phase=0  t230_QT_dac2_coarse_freq=0  t230_QT_dac2_nyquist_zone=Zone 1  t230_QT_dac2_decode_mode=SNR Optimized  t230_QT_dac3_enable=off  t230_QT_dac3_analog_output=Real  t230_QT_dac3_inter_mode=4x  t230_QT_dac3_sample_per_cycle=2  t230_QT_dac3_req_axis_clk=250  t230_QT_dac3_datapath_mode=DUC 0 to Fs/2  t230_QT_dac3_mixer_type=Bypassed  t230_QT_dac3_mixer_mode=Real -> Real  t230_QT_dac3_nco_freq=0  t230_QT_dac3_nco_phase=0  t230_QT_dac3_coarse_freq=0  t230_QT_dac3_nyquist_zone=Zone 1  t230_QT_dac3_decode_mode=SNR Optimized  Tile231_enable=off  t231_enable_mts=off  t231_sample_rate=2000  t231_clk_out=125  t231_enable_pll=on  t231_ref_clk=250  t231_output_power=20  t231_QT_dac0_enable=on  t231_QT_dac0_analog_output=Real  t231_QT_dac0_inter_mode=4x  t231_QT_dac0_sample_per_cycle=2  t231_QT_dac0_req_axis_clk=250  t231_QT_dac0_datapath_mode=DUC 0 to Fs/2  t231_QT_dac0_mixer_type=Bypassed  t231_QT_dac0_mixer_mode=Real -> Real  t231_QT_dac0_nco_freq=0  t231_QT_dac0_nco_phase=0  t231_QT_dac0_coarse_freq=0  t231_QT_dac0_nyquist_zone=Zone 1  t231_QT_dac0_decode_mode=SNR Optimized  t231_QT_dac1_enable=off  t231_QT_dac1_analog_output=Real  t231_QT_dac1_inter_mode=4x  t231_QT_dac1_sample_per_cycle=2  t231_QT_dac1_req_axis_clk=250  t231_QT_dac1_datapath_mode=DUC 0 to Fs/2  t231_QT_dac1_mixer_type=Bypassed  t231_QT_dac1_mixer_mode=Real -> Real  t231_QT_dac1_nco_freq=0  t231_QT_dac1_nco_phase=0  t231_QT_dac1_coarse_freq=0  t231_QT_dac1_nyquist_zone=Zone 1  t231_QT_dac1_decode_mode=SNR Optimized  t231_QT_dac2_enable=off  t231_QT_dac2_analog_output=Real  t231_QT_dac2_inter_mode=4x  t231_QT_dac2_sample_per_cycle=2  t231_QT_dac2_req_axis_clk=250  t231_QT_dac2_datapath_mode=DUC 0 to Fs/2  t231_QT_dac2_mixer_type=Bypassed  t231_QT_dac2_mixer_mode=Real -> Real  t231_QT_dac2_nco_freq=0  t231_QT_dac2_nco_phase=0  t231_QT_dac2_coarse_freq=0  t231_QT_dac2_nyquist_zone=Zone 1  t231_QT_dac2_decode_mode=SNR Optimized  t231_QT_dac3_enable=off  t231_QT_dac3_analog_output=Real  t231_QT_dac3_inter_mode=4x  t231_QT_dac3_sample_per_cycle=2  t231_QT_dac3_req_axis_clk=250  t231_QT_dac3_datapath_mode=DUC 0 to Fs/2  t231_QT_dac3_mixer_type=Bypassed  t231_QT_dac3_mixer_mode=Real -> Real  t231_QT_dac3_nco_freq=0  t231_QT_dac3_nco_phase=0  t231_QT_dac3_coarse_freq=0  t231_QT_dac3_nyquist_zone=Zone 1  t231_QT_dac3_decode_mode=SNR Optimized  t224_has_adc_clk=on  t224_adc_clk_src=224  t224_clk_dist=Input Refclk  t225_has_adc_clk=off  t225_adc_clk_src=224  t225_clk_dist=None  t226_has_adc_clk=on  t226_adc_clk_src=226  t226_clk_dist=Input Refclk  t227_has_adc_clk=off  t227_adc_clk_src=226  t227_clk_dist=None  t228_has_dac_clk=on  t228_dac_clk_src=228  t228_clk_dist=Input Refclk  t229_has_dac_clk=off  t229_dac_clk_src=228  t229_clk_dist=None  t230_has_dac_clk=on  t230_dac_clk_src=230  t230_clk_dist=Input Refclk  t231_has_dac_clk=off  t231_dac_clk_src=230  t231_clk_dist=None  maskdoneopening=0
      settings: SourceProductName=CASPER XPS Blockset
  slice_enable : xbsIndex_r4/Slice  nbits=1  boolean_output=on  mode=Lower Bit Location + Width  bit1=0  base1=MSB of Input  bit0=0  base0=LSB of Input  dbl_ovrd=off  block_type=slice
  slice_msb : xbsIndex_r4/Slice  nbits=1  boolean_output=off  mode=Upper Bit Location + Width  bit1=0  base1=MSB of Input  bit0=0  base0=LSB of Input  dbl_ovrd=off  block_type=slice
  slice_reset : xbsIndex_r4/Slice  nbits=1  boolean_output=on  mode=Lower Bit Location + Width  bit1=0  base1=MSB of Input  bit0=1  base0=LSB of Input  dbl_ovrd=off  block_type=slice
  snapshot_ctrl : Subsystem  Tag=xps:sw_reg  AncestorBlock=xps_library/Memory/software_register  mask(swreg){io_dir=From Processor, io_delay=0, init_val=0, sample_period=1, names=[start], bitwidths=1, bin_pts=0, arith_types=2, sim_port=on, show_format=on}
      mask prompts: io_dir "I/O direction"; io_delay "I/O delay"; init_val "Initial Value"; sample_period "Sample period"; names "Bitfield names [msb...lsb]"; bitwidths "Bitfield widths"; bin_pts "Bitfield binary pts"; arith_types "Bitfield types, ufix=0, fix=1, bool=2"; sim_port "Provide sim input/output?"; show_format "Print format string?"
      mask help: A 32-bit software-accessible register. Can be divided into bitfields of varying widths and types using the fields in the block mask.
      mask init:
      | swreg_init(gcb)
      settings: AttributesFormatString=1input:b = 1 bits
      mask TypeOptions io_dir: To Processor | From Processor
      mask Callback io_dir:
      | mask_enables = get_param(gcb, 'MaskEnables');
      | mask_names = get_param(gcb, 'MaskNames');
      | if strcmp(get_param(gcb, 'io_dir'), 'To Processor'),
      |     mask_enables{ismember(mask_names, 'sample_period')} = 'off';
      | else
      |     mask_enables{ismember(mask_names, 'sample_period')} = 'on';
      | end
      | set_param(gcb, 'MaskEnables', mask_enables);
      mask DialogControl ParameterTabVar0 Prompt: Setup
  sum_a_b : Subsystem  Tag=xps:sw_reg  AncestorBlock=xps_library/Memory/software_register  mask(swreg){io_dir=To Processor, io_delay=0, init_val=0, sample_period=1, names=reg, bitwidths=32, bin_pts=0, arith_types=0, sim_port=on, show_format=off}
      mask prompts: io_dir "I/O direction"; io_delay "I/O delay"; init_val "Initial Value"; sample_period "Sample period"; names "Bitfield names [msb...lsb]"; bitwidths "Bitfield widths"; bin_pts "Bitfield binary pts"; arith_types "Bitfield types, ufix=0, fix=1, bool=2"; sim_port "Provide sim input/output?"; show_format "Print format string?"
      mask help: A 32-bit software-accessible register. Can be divided into bitfields of varying widths and types using the fields in the block mask.
      mask init:
      | swreg_init(gcb)
      settings: AttributesFormatString=1output
      mask TypeOptions io_dir: To Processor | From Processor
      mask Callback io_dir:
      | mask_enables = get_param(gcb, 'MaskEnables');
      | mask_names = get_param(gcb, 'MaskNames');
      | if strcmp(get_param(gcb, 'io_dir'), 'To Processor'),
      |     mask_enables{ismember(mask_names, 'sample_period')} = 'off';
      | else
      |     mask_enables{ismember(mask_names, 'sample_period')} = 'on';
      | end
      | set_param(gcb, 'MaskEnables', mask_enables);
      mask DialogControl ParameterTabVar0 Prompt: Setup
  wires:
  slice_enable/1 -> counter_led1/2
  gpio/1(sim_out) -> Terminator/1
  slice_reset/1 -> counter_led1/1
  sum_a_b/1(sim_out_reg) -> Scope1/1
  b_sim/1 -> bin/1(sim_1)
  counter_led/1 -> slice_msb/1
  counter_led1/1 -> counter_value/1(out_reg)
  counter_ctrl/1(in_reg) -> slice_reset/1, slice_enable/1
  counter_value/1(sim_out_reg) -> Scope/1
  Constant/1 -> counter_ctrl/1(sim_1)
  AddSub/1 -> sum_a_b/1(out_reg)
  rfdc/1 -> bitfield_snapshot/1(in_m00)
  ain/1(in_reg) -> AddSub/1
  a_sim/1 -> ain/1(sim_1)
  Constant4/1 -> snapshot_ctrl/1(sim_1)
  snapshot_ctrl/1(in_start) -> edge_detect1/1
  slice_msb/1 -> Inverter/1
  Inverter/1 -> gpio/1(gpio_out)
  bin/1(in_reg) -> AddSub/2
  rfdc/7 -> bitfield_snapshot2/1(in_m20)
  rfdc/3 -> bitfield_snapshot1/1(in_m02)
  rfdc/9 -> bitfield_snapshot3/1(in_m22)
  rfdc/2 -> bitfield_snapshot/2(in_m01)
  rfdc/4 -> bitfield_snapshot1/2(in_m03)
  rfdc/8 -> bitfield_snapshot2/2(in_m21)
  rfdc/10 -> bitfield_snapshot3/2(in_m23)
  edge_detect1/1 -> bitfield_snapshot/4(trig), bitfield_snapshot2/4(trig), bitfield_snapshot1/4(trig), bitfield_snapshot3/4(trig)
  Constant1/1 -> bitfield_snapshot/3(we), bitfield_snapshot1/3(we), bitfield_snapshot2/3(we), bitfield_snapshot3/3(we)

== system rfsoc4x2_tut_rfdc/RFSoC4x2 ==

== system rfsoc4x2_tut_rfdc/ain ==
  sim_1 : Inport
  convert1_1 : DataTypeConversion  OutDataTypeStr=fixdt('ufix32_En0')  LockScale=on
  convert2_1 : DataTypeConversion  OutDataTypeStr=fixdt('ufix32_En0')  ConvertRealWorld=Stored Integer (SI)  LockScale=on
  gain_1 : Gain
  io_delay : xbsIndex_r4/Delay  rst=off  infoeditControl=Selection of Reset will increase slice count due to use of real FFs and instead of SRLs  en=off  latency=0  reg_retiming=on  dbl_ovrd=off  block_type=delay
  reint1 : xbsIndex_r4/Reinterpret  force_arith_type=on  arith_type=Unsigned  force_bin_pt=on  bin_pt=0  block_type=reinterpret
  rfsoc4x2_tut_rfdc_ain_user_data_out : xbsIndex_r4/Gateway In  gui_display_data_type=Fixed-point  arith_type=Unsigned  n_bits=32  bin_pt=0  preci_type=Single  exp_width=8  frac_width=24  rows=1  columns=1  quantization="Round  (unbiased: +/- Inf)"  overflow=Saturate  period=1  UseAsADC=off  ADCChannel='1'  interface=None  automatic_assignment=on  address_offset=hex2dec('00')  intf_name=''  intf_description=''  default_value=0  timing_constraint=None  locs_specified=off  LOCs={}  io_standard={}  inherit_from_input=off  hdl_port=on  dbl_ovrd=off  block_type=gatewayin
  slice_reg : xbsIndex_r4/Slice  nbits=32  boolean_output=off  mode=Lower Bit Location + Width  bit1=0  base1=MSB of Input  bit0=0  base0=LSB of Input  dbl_ovrd=off  block_type=slice
  in_reg : Outport
  wires:
  rfsoc4x2_tut_rfdc_ain_user_data_out/1 -> io_delay/1
  sim_1/1 -> convert1_1/1
  convert1_1/1 -> convert2_1/1
  convert2_1/1 -> gain_1/1
  gain_1/1 -> rfsoc4x2_tut_rfdc_ain_user_data_out/1
  io_delay/1 -> slice_reg/1
  slice_reg/1 -> reint1/1
  reint1/1 -> in_reg/1
